simulink model "automaticWiperController_Harness1"  (R2024b)
settings: Solver=VariableStepAuto  StartTime=0.0  StopTime=20  RelTol=1e-3
libraries: SignalEditorBlockLib x1
settings Model: Creator=ACER  LastModifiedBy=ACER
settings ConfigComp: CovEnable=on  CovScope=ReferencedModels  CovIncludeTopModel=off  CovMetricSettings=dcmwe  CovEnableCumulative=off  CovModelRefEnable=on

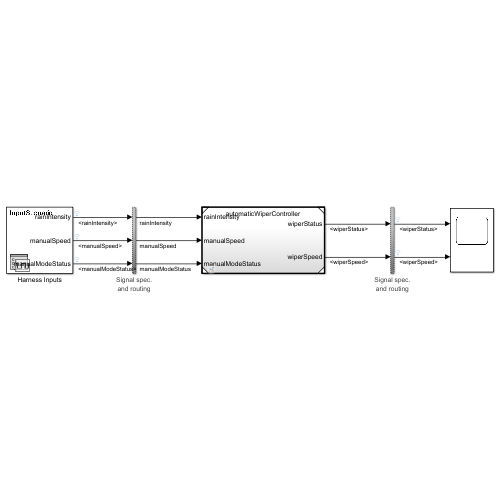
[thumbnail: Simulink's stored preview of the top-level diagram]
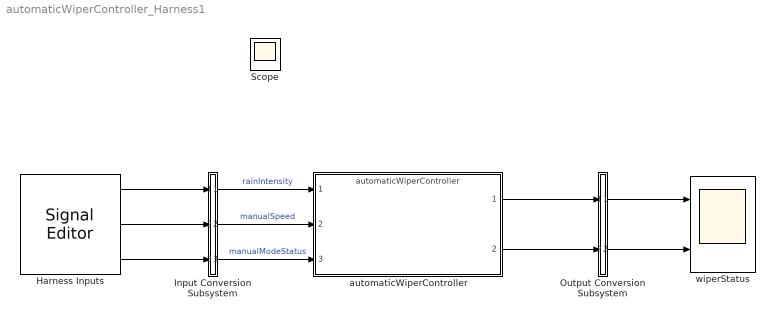
== system automaticWiperController_Harness1 ==
  Harness Inputs : SignalEditorBlockLib/Signal Editor  FileName=automaticWiperController_Harness1_HarnessInputs_1.mat  ActiveScenario=InputScenario  ActiveSignal=manualModeStatus  IsBus=off  OutputBusObjectStr=Bus: BusObject  SampleTime=0.01  Interpolate=off  ZeroCross=off  OutputAfterFinalValue=Setting to zero  Unit=inherit  PreserveSignalName=on  ApplySigPropsToAllScenarios=on  ApplySigPropsToAllSignals=on
  Input Conversion Subsystem : Subsystem  Tag=__SLT_ICS__  Description=|
      | Signal spec.
      | and routing
      settings: AttributesFormatString=%<Description>
  Output Conversion Subsystem : Subsystem  Tag=__SLT_OCS__  Description=|
      | Signal spec.
      | and routing
      settings: AttributesFormatString=%<Description>
  automaticWiperController : ModelReference  ModelNameDialog=automaticWiperController  SimulationMode=Normal  ModelReferenceVersion=1.24
  wiperStatus : Scope  NumInputPorts=2
  Scope : Scope
  wires:
  Harness Inputs/1 -> Input Conversion Subsystem/1(Inport_1)
  Harness Inputs/2 -> Input Conversion Subsystem/2(Inport_2)
  Harness Inputs/3 -> Input Conversion Subsystem/3(Inport_3)
  Output Conversion Subsystem/1(Outport_1) -> wiperStatus/1
  Output Conversion Subsystem/2(Outport_2) -> wiperStatus/2
  Input Conversion Subsystem/1(Outport_1) -> automaticWiperController/1  "rainIntensity"
  Input Conversion Subsystem/2(Outport_2) -> automaticWiperController/2  "manualSpeed"
  Input Conversion Subsystem/3(Outport_3) -> automaticWiperController/3  "manualModeStatus"
  automaticWiperController/1 -> Output Conversion Subsystem/1(Inport_1)
  automaticWiperController/2 -> Output Conversion Subsystem/2(Inport_2)

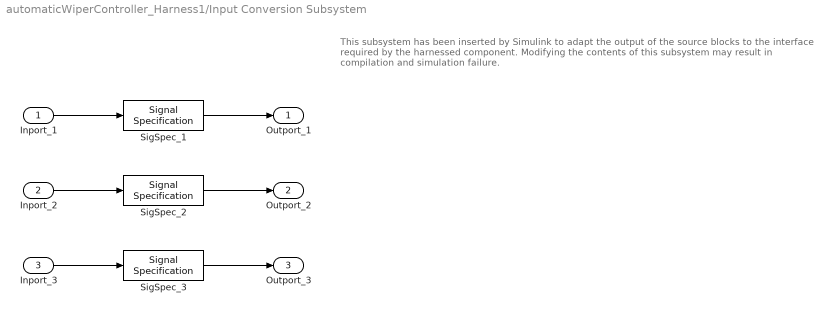
== system automaticWiperController_Harness1/Input Conversion Subsystem ==
  note: This subsystem has been inserted by Simulink to adapt the output of the source blocks to the interface required by the harnessed component.
      |  Modifying the contents of this subsystem may result in compilation and simulation failure.
  Inport_1 : Inport
  Inport_2 : Inport  Port=2
  Inport_3 : Inport  Port=3
  SigSpec_1 : SignalSpecification  OutDataTypeStr=Enum: intensityEnum  Dimensions=[1]  SampleTime=0.01
  SigSpec_2 : SignalSpecification  OutDataTypeStr=Enum: intensityEnum  Dimensions=[1]  SampleTime=0.01
  SigSpec_3 : SignalSpecification  OutDataTypeStr=Enum: onOffEnum  Dimensions=[1]  SampleTime=0.01
  Outport_1 : Outport
  Outport_2 : Outport  Port=2
  Outport_3 : Outport  Port=3
  wires:
  SigSpec_1/1 -> Outport_1/1
  Inport_1/1 -> SigSpec_1/1
  SigSpec_2/1 -> Outport_2/1
  Inport_2/1 -> SigSpec_2/1
  SigSpec_3/1 -> Outport_3/1
  Inport_3/1 -> SigSpec_3/1

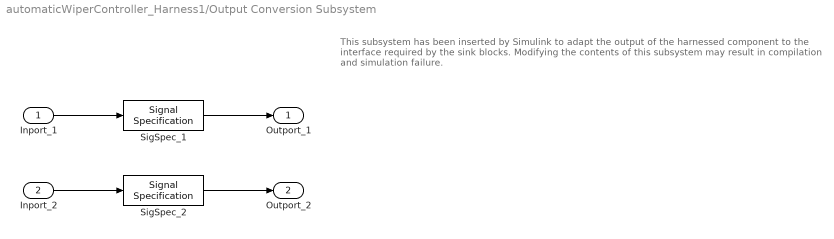
== system automaticWiperController_Harness1/Output Conversion Subsystem ==
  note: This subsystem has been inserted by Simulink to adapt the output of the harnessed component to the interface required by the sink blocks.
      |  Modifying the contents of this subsystem may result in compilation and simulation failure.
  Inport_1 : Inport
  Inport_2 : Inport  Port=2
  SigSpec_1 : SignalSpecification  OutDataTypeStr=Enum: onOffEnum  Dimensions=[1]  SampleTime=0.01
  SigSpec_2 : SignalSpecification  OutDataTypeStr=Enum: wiperSpeedEnum  Dimensions=[1]  SampleTime=0.01
  Outport_1 : Outport
  Outport_2 : Outport  Port=2
  wires:
  Inport_1/1 -> SigSpec_1/1
  SigSpec_1/1 -> Outport_1/1
  Inport_2/1 -> SigSpec_2/1
  SigSpec_2/1 -> Outport_2/1
